simulink model "aaa"  (R2023a)
settings: Solver=VariableStepAuto  StartTime=0.0  StopTime=200  RelTol=1e-3
model workspace (MAT data in the model file):
  Queries_MAX = 100
  Task_Weight = 2
  Threshold_Val = 0.1
  lambda = 0.25
values from neighbouring files (symbols this model uses):
  m = m + 1    (= 2)    [TMO5liubimov.m]    (also in laba2.m = 14; laba3.m = 200; test.m = 5)
  n = 31    [laba2.m]    (also in test.m = 7)
libraries: slrealtimeloglib x16
settings Model: PacingRate=501  Creator=error  LastModifiedBy=PC

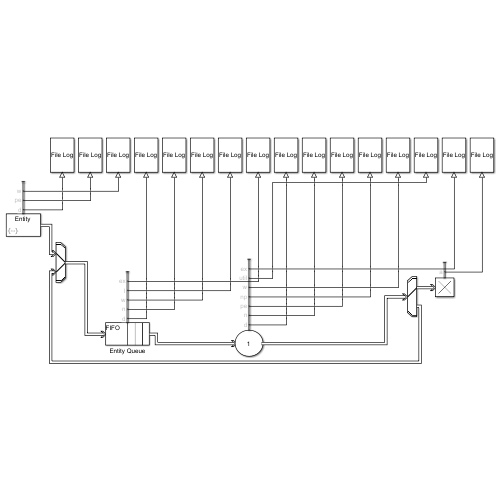
[thumbnail: Simulink's stored preview of the top-level diagram]
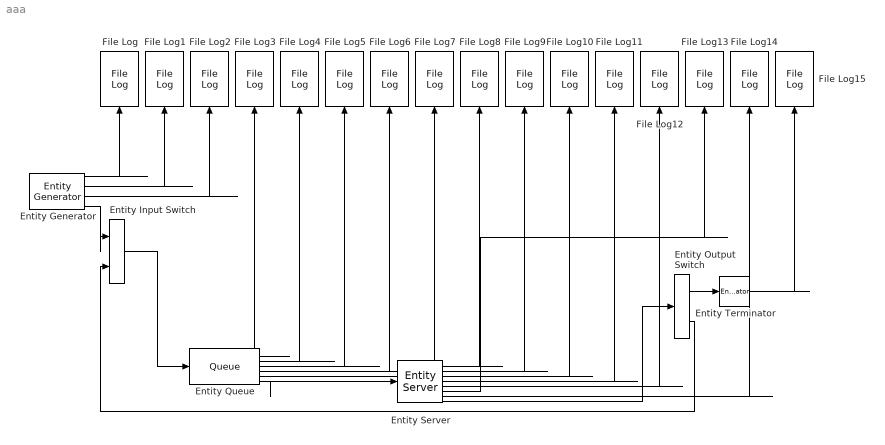
== system aaa ==
  Entity Input Switch : EntityInputSwitch  InputPortMessageModes=m,m  OutputPortMessageModes=m
  Entity Output Switch : EntityOutputSwitch  InputPortMessageModes=m  OutputPortMessageModes=m,m  SwitchingCriterion=From attribute  SwitchAttributeName=reject
  Entity Generator : EntityGenerator  OutputPortMessageModes=n,n,n,m  TimeSource=MATLAB action  IntergenerationTimeAction=|  GenerateAction=entity.reject = randi([1, 2]);  AttributeName=weight|reject  AttributeInitialValue=1|1  NumberEntitiesDeparted=on  PendingEntityInBlock=on  AverageIntergenerationTime=on  EntityType=Structured  EntityTypeName=Entity
      | persistent n;
      | if isempty(n)
      |     n = 0;
      | end
      | n = n + 1;
      | 
      | if n <= Queries_MAX
      |     dt = exprnd(1/lambda);
      | else
      |     dt = inf;
      | end
      settings: OutputPortMap=o0,o1,o2,o3
  Entity Queue : Queue  InputPortMessageModes=m  OutputPortMessageModes=n,n,n,n,n,m  NumberEntitiesDeparted=on  NumEntitiesExtracted=on  NumberEntitiesInBlock=on  AverageWait=on  AverageQueueLength=on
      settings: OutputPortMap=o0,o1,o2,o3,o7,o5
  Entity Server : EntityServer  InputPortMessageModes=m  OutputPortMessageModes=n,n,n,n,n,n,n,m  Capacity=1  ServiceTimeSource=MATLAB action  ServiceTimeAction=dt = rand(1,1) + entity.weight;  NumberEntitiesDeparted=on  NumberEntitiesInBlock=on  PendingEntityPresentInBlock=on  NumberEntitiesPending=on  AverageWait=on  Utilization=on  NumEntitiesExtracted=on
      settings: OutputPortMap=o0,o1,o2,o3,o4,o5,o12,o9
  Entity Terminator : EntityTerminator  InputPortMessageModes=m  NumberEntitiesArrived=on
      settings: OutputPortMap=o0
  File Log{,1..15} (16 alike) : slrealtimeloglib/File Log  decimation=1  inputProcessing=Elements as channels (sample based)
  wires:
  Entity Generator/4 -> Entity Input Switch/1
  Entity Input Switch/1 -> Entity Queue/1
  Entity Queue/6 -> Entity Server/1
  Entity Server/8 -> Entity Output Switch/1
  Entity Output Switch/2 -> Entity Input Switch/2
  Entity Output Switch/1 -> Entity Terminator/1
  Entity Generator/1 -> File Log/1
  Entity Generator/2 -> File Log1/1
  Entity Generator/3 -> File Log2/1
  Entity Queue/1 -> File Log3/1
  Entity Queue/2 -> File Log4/1
  Entity Queue/3 -> File Log5/1
  Entity Queue/4 -> File Log6/1
  Entity Queue/5 -> File Log7/1
  Entity Server/1 -> File Log8/1
  Entity Server/2 -> File Log9/1
  Entity Server/3 -> File Log10/1
  Entity Server/4 -> File Log11/1
  Entity Server/5 -> File Log12/1
  Entity Server/6 -> File Log13/1
  Entity Server/7 -> File Log14/1
  Entity Terminator/1 -> File Log15/1
